simulink model "Problem1_b"  (Simulink 7.5)
settings: Solver=ode45  StartTime=0.0  StopTime=10.0  RelTol=1e-3
libraries: simulink x1
settings Model: Creator=m.bagheri1986  LastModifiedBy=m.bagheri1986

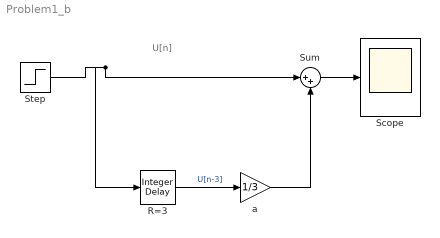
== system Problem1_b ==
  note: U[n]
  "R=3 " : simulink/Discrete/Integer Delay  vinit=0.0  samptime=-1  NumDelays=3
  Scope : Scope
  Step : Step  Time=1/10  Before=1  After=0  SampleTime=1/10
  Sum : Sum  Inputs=|++  OutDataType=fixdt(1, 16)  OutScaling=2^0
  a : Gain  Gain=1/3  ParameterDataType=fixdt(1, 16)  ParameterScaling=2^0  OutDataType=fixdt(1, 16)  OutScaling=2^0
  wires:
  "R=3 "/1 -> a/1  "U[n-3]"
  Sum/1 -> Scope/1
  Step/1 -> "R=3 "/1, Sum/1
  a/1 -> Sum/2
